simulink model "analysis_lateral_accelration"  (R2019b)
settings: Solver=VariableStepAuto  StartTime=0.0  StopTime=10.0  RelTol=1e-3
values from neighbouring files (symbols this model uses):
  a0 = a11.*a22 - a12.*a21    [coefficien_lateral_accelration.m]    (also in coefficien_sideslip_angre.m; coefficien_turning_trajectory.m; coefficien_yawrate.m)
  a1 = -a11-a22    [coefficien_lateral_accelration.m]    (also in coefficien_sideslip_angre.m; coefficien_turning_trajectory.m; coefficien_yawrate.m)
  b0 = a21.*b11 - a11.*b21    [coefficien_lateral_accelration.m]    (also in coefficien_sideslip_angre.m = a12.*b21 - a22.*b11; coefficien_turning_trajectory.m; coefficien_yawrate.m)
  b1 = a12.*b21 - a22.*b11 + b21    [coefficien_lateral_accelration.m]    (also in coefficien_sideslip_angre.m = b11; coefficien_turning_trajectory.m; coefficien_yawrate.m = b21)
  b2 = b11    [coefficien_lateral_accelration.m]    (also in coefficien_turning_trajectory.m)
  V = [8.33333333333 16.6666666667 25 33.3333333333 41.6666666667 50]    [block_params.mat]    (also in coefficien.m = [30:30:180]/3.6; coefficien_lateral_accelration.m = V*(1000/(60*60)); coefficien_sideslip_angre.m = V*(1000/(60*60)); coefficien_turning_trajectory.m = V*(1000/(60*60)))
libraries: cstblocks x1
settings Model: Creator=Natsu Nakagawa  LastModifiedBy=Natsu Nakagawa

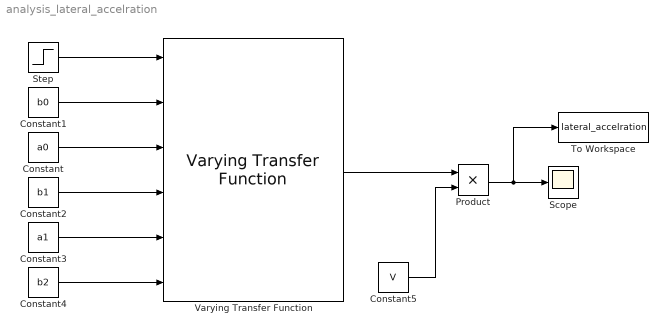
== system analysis_lateral_accelration ==
  Constant : Constant  Value=a0
  Constant1 : Constant  Value=b0
  Constant2 : Constant  Value=b1
  Constant3 : Constant  Value=a1
  Constant4 : Constant  Value=b2
  Constant5 : Constant  Value=V
  Product : Product
  Scope : Scope
  Step : Step  Time=0  SampleTime=0
  To Workspace : ToWorkspace  VariableName=lateral_accelration  SaveFormat=Timeseries  SampleTime=-1
  Varying Transfer Function : cstblocks/Linear Parameter Varying/Varying Transfer Function  N=2
      settings: SourceProductName=Control System Toolbox
  wires:
  Constant4/1 -> Varying Transfer Function/6
  Varying Transfer Function/1 -> Product/1
  Constant3/1 -> Varying Transfer Function/5
  Constant1/1 -> Varying Transfer Function/2
  Constant2/1 -> Varying Transfer Function/4
  Constant/1 -> Varying Transfer Function/3
  Step/1 -> Varying Transfer Function/1
  Constant5/1 -> Product/2
  Product/1 -> To Workspace/1, Scope/1
